simulink model "ESTS_TFY_YawMomFromFx_test"  (R2023b)
settings: Solver=VariableStepAuto  StartTime=0.0  StopTime=10.0  RelTol=1e-3
libraries: ESTS_TFY_YawMomFromFx x1
settings Model: Creator=blatak  LastModifiedBy=blatak

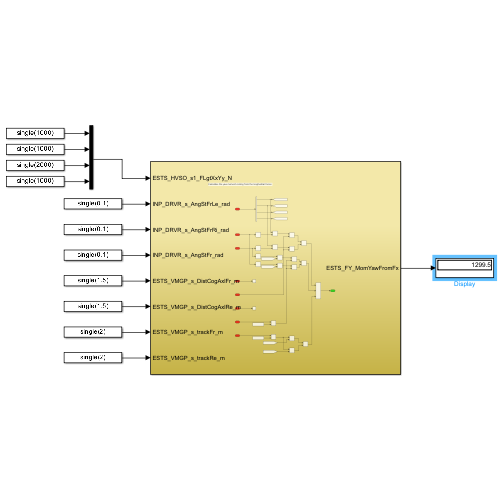
[thumbnail: Simulink's stored preview of the top-level diagram]
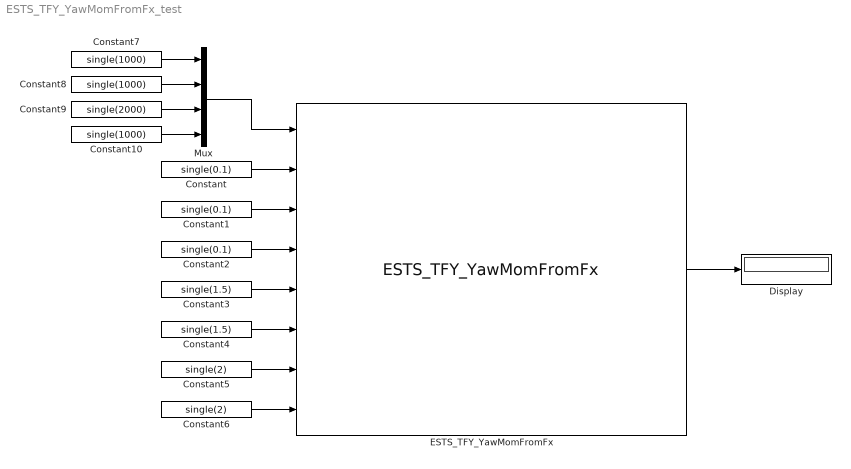
== system ESTS_TFY_YawMomFromFx_test ==
  Constant : Constant  Value=single(0.1)
  Constant1 : Constant  Value=single(0.1)
  Constant10 : Constant  Value=single(1000)
  Constant2 : Constant  Value=single(0.1)
  Constant3 : Constant  Value=single(1.5)
  Constant4 : Constant  Value=single(1.5)
  Constant5 : Constant  Value=single(2)
  Constant6 : Constant  Value=single(2)
  Constant7 : Constant  Value=single(1000)
  Constant8 : Constant  Value=single(1000)
  Constant9 : Constant  Value=single(2000)
  Display : Display
  ESTS_TFY_YawMomFromFx : ESTS_TFY_YawMomFromFx/ESTS_TFY_YawMomFromFx  SystemSampleTime=-1  VariantActivationTime=update diagram  AllowFlexibleInterface=on  Latency=0  AutoFrameSizeCalculation=off
  Mux : Mux
  wires:
  Constant/1 -> ESTS_TFY_YawMomFromFx/2
  Constant7/1 -> Mux/1
  Constant8/1 -> Mux/2
  Constant9/1 -> Mux/3
  Constant10/1 -> Mux/4
  Mux/1 -> ESTS_TFY_YawMomFromFx/1
  Constant1/1 -> ESTS_TFY_YawMomFromFx/3
  Constant2/1 -> ESTS_TFY_YawMomFromFx/4
  Constant3/1 -> ESTS_TFY_YawMomFromFx/5
  Constant4/1 -> ESTS_TFY_YawMomFromFx/6
  Constant5/1 -> ESTS_TFY_YawMomFromFx/7
  Constant6/1 -> ESTS_TFY_YawMomFromFx/8
  ESTS_TFY_YawMomFromFx/1 -> Display/1
